simulink model "Book4342"  (R2019b)
settings: Solver=ode4  StartTime=0  StopTime=30  FixedStep=0.001  RelTol=1e-3
settings Model: Creator=xyh  LastModifiedBy=user

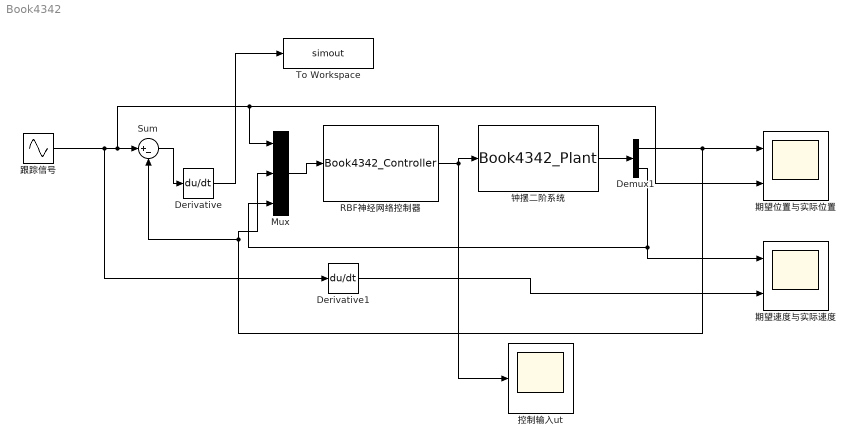
== system Book4342 ==
  Demux1 : Demux  Outputs=2
  Derivative : Derivative
  Derivative1 : Derivative
  Mux : Mux  Inputs=3
  RBF神经网络控制器 : S-Function  FunctionName=Book4342_Controller  SFunctionDeploymentMode=off  EnableBusSupport=off
  Sum : Sum  Inputs=|+-
  To Workspace : ToWorkspace  VariableName=simout  SaveFormat=Timeseries  SampleTime=-1
  控制输入ut : Scope
  期望位置与实际位置 : Scope  NumInputPorts=2
  期望速度与实际速度 : Scope  NumInputPorts=2
  跟踪信号 : Sin  Amplitude=pi/6  SampleTime=0
  钟摆二阶系统 : S-Function  FunctionName=Book4342_Plant  SFunctionDeploymentMode=off  EnableBusSupport=off
  wires:
  Mux/1 -> RBF神经网络控制器/1
  RBF神经网络控制器/1 -> 钟摆二阶系统/1, 控制输入ut/1
  跟踪信号/1 -> Derivative1/1, Sum/1, Mux/1, 期望位置与实际位置/2
  Derivative1/1 -> 期望速度与实际速度/2
  钟摆二阶系统/1 -> Demux1/1
  Sum/1 -> Derivative/1
  Demux1/1 -> 期望位置与实际位置/1, Mux/2, Sum/2
  Demux1/2 -> Mux/3, 期望速度与实际速度/1
  Derivative/1 -> To Workspace/1
